simulink model "Exp1"  (R2025b)
settings: Solver=VariableStepAuto  StartTime=0.0  StopTime=10.0  RelTol=1e-3
libraries: simulink x1
settings Model: Creator=pc  LastModifiedBy=pc

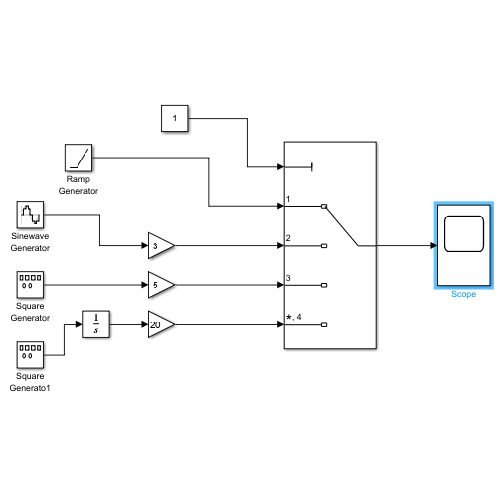
[thumbnail: Simulink's stored preview of the top-level diagram]
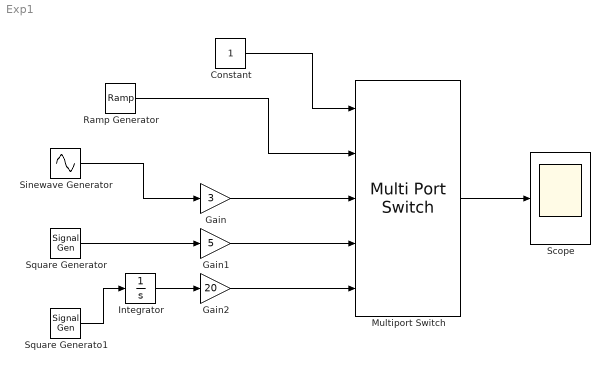
== system Exp1 ==
  Constant : Constant
  Gain : Gain  Gain=3
  Gain1 : Gain  Gain=5
  Gain2 : Gain  Gain=20
  Integrator : Integrator
  Multiport Switch : MultiPortSwitch  Inputs=4  SaturateOnIntegerOverflow=off  InputSameDT=off
  Ramp Generator : simulink/Sources/Ramp  slope=1  start=0  InitialOutput=0
  Scope : Scope
      settings: ActiveDisplayYMinimum=-1.2499999999999998  ActiveDisplayYMaximum=11.25
  "Sinewave Generator " : Sin  Frequency=2*pi  SampleTime=1/10000
  Square Generato1 : SignalGenerator  WaveForm=square  Frequency=2*pi  Units=rad/sec
  Square Generator : SignalGenerator  WaveForm=square  Frequency=2*pi  Units=rad/sec
  wires:
  Ramp Generator/1 -> Multiport Switch/2
  Constant/1 -> Multiport Switch/1
  "Sinewave Generator "/1 -> Gain/1
  Gain/1 -> Multiport Switch/3
  Square Generator/1 -> Gain1/1
  Gain1/1 -> Multiport Switch/4
  Square Generato1/1 -> Integrator/1
  Integrator/1 -> Gain2/1
  Gain2/1 -> Multiport Switch/5
  Multiport Switch/1 -> Scope/1
